simulink model "P300_directions"  (R2012b)
settings: Solver=VariableStepDiscrete  StartTime=0.0  StopTime=5000  FixedStep=1/256  RelTol=1e-3
InitFcn:
  | clear global handle
  | 
  | clear global userData
  | 
  | if exist('P300classifier') ~=1
  | global P300classifier
  | P300classifier.method = 0;
  | end
undefined symbols (not defined in the file): THblink, THfrown, THgazeL, THgazeR, THwinkL, THwinkR
libraries: dspsigops x4, dspstat3 x2, gtecHighspeedLib x2
settings Model: Creator=Markus Waldhauser  LastModifiedBy=MA
settings DataIOCC: SignalLoggingSaveFormat=ModelDataLogs
settings OptimizationCC: InitFltsAndDblsToZero=on
settings DebuggingCC: SaveWithParameterizedLinksMsg=none  SignalResolutionControl=TryResolveAllWithWarning  MultiTaskDSMMsg=warning  MultiTaskCondExecSysMsg=none  FcnCallInpInsideContextMsg=UseLocalSettings  StrictBusMsg=Warning
settings RTWCC: IncludeERTFirstTime=on
settings GRTTargetCC: TargetFcnLib=ansi_tfl_tmw.mat  CombineOutputUpdateFcns=off  GRTInterface=on

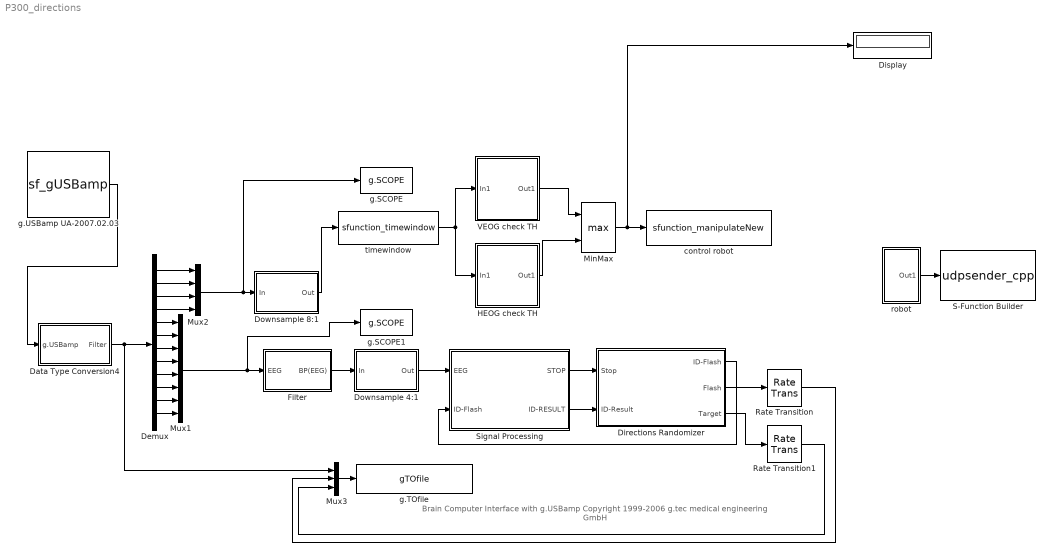
== system P300_directions ==
  note: Brain Computer Interface with g.USBamp
      | Copyright 1999-2006 g.tec medical engineering GmbH
  Data Type Conversion4 : Subsystem
  Demux : Demux  Outputs=12
  Directions Randomizer : Subsystem  mask(Single Character Flash Speller){mode=Free Ride, flashtime=100, darktime=100}
      mask prompts: flashtime "Flash time [ms]:"; darktime "Dark time [ms]:"
      mask help: Displays a 36 character matrix. Each character is flashing up for a specific time in a random and sequential order. The dark time is the time between the characters.
      mask init:
      | set_param('P300_directions/Directions Randomizer/StopSimu','Gain','0');
      | set_param('P300_directions/Directions Randomizer/Switch','Gain','0');
      mask Help:
      | Displays a 36 character matrix. Each character is flashing up for a specific time in a random and sequential order. The dark time is the time between the characters. If the character is flashing up the ID-Flash is transmitted for the Signal Processing. Flash contains the ID of every character. Target is one if a specific character for the copy spelling mode flashes up. <br><br>
      | 
      | Mode - can be Copy Spelling or Free Spelling<br><br>
      | Flash time [ms] - time that character is shown on screen <br><br>
      | Dark time [ms] - time between the characters
      mask TypeOptions mode: Copy Ride | Free Ride
      mask Display:
      | image(imread('dirs.png'))
      | port_label('output',1,'ID-Flash')
      | port_label('output',2,'Flash')
      | port_label('output',3,'Target')
      | port_label('input',1,'Stop')
      | port_label('input',2,'ID')
  Display : Display
      mask Display: disp('D blink');
  Downsample 4:1 : Subsystem
  Downsample 8:1 : Subsystem
  Filter : Subsystem  Tag=FilterWizardSubSystem
      settings: ErrorFcn=dspFilterRealizedInBasicElemsAlgLoopErrFcnCallback
  HEOG check TH : Subsystem
  MinMax : MinMax  Function=max  Inputs=2
  Mux1 : Mux  Inputs=8
  Mux2 : Mux
  Mux3 : Mux  Inputs=3
  Rate Transition : RateTransition
  Rate Transition1 : RateTransition
  S-Function Builder : S-Function  InitFcn=try, set_param(gcb,'FunctionName','udpsender_cpp'), end  FunctionName=udpsender_cpp  Parameters=int32(1)  SFunctionModules=udpsender_cpp_wrapper  EnableBusSupport=off  mask(S-Function Builder){}
      mask help: Simulink:masks:SFunctionBuilder_MD
      mask init:
      | val = [[.9  0.75 0.75 1 1 .9 .9 1]',[1 1 0.75 0.75 .9 .9 1 .9]'];try , sys = get_param(gcb,'SfunBuilderFcnName');if isempty(sys), sys = get_param(gcb,'FunctionName'); end,catch, sys = get_param(gcb,'FunctionName'); end
      settings: CopyFcn=set_param(gcbh,'LinkStatus','none')  PreSaveFcn=try, set_param(gcb,'FunctionName','udpsender_cpp'), end  OpenFcn=sfunctionwizard(gcbh)
      mask Display: plot(val(:,1),val(:,2)),disp(sys), port_label('input',1,'u0')
  Signal Processing : Subsystem  mask(P300 Signal Processing){windTime=800, runmax=2, channels=8, method=Linear Discriminant Analysis}
      mask prompts: windTime "Buffer length [ms]"; runmax "Number of flashes:"; channels "Number of channels:"; method "Classification Method:"
      mask help: The block buffers EEG data for each ID-Flash obtained. As soon as M (Number of flashes) characters of each ID are obtained a STOP command is sent and the maximum P300 is calculated and applied on output ID.
      mask Help:
      | P300 Signal Processing block. The block buffers EEG data for each ID-Flash obtained. As soon as M (Number of flashes) characters of each ID are obtained a STOP command is sent. Then the maximum P300 is calculated and the character ID is sent. <br><br>
      | 
      | Buffer length [ms] - enter the EEG data buffer size <br><br>
      | Number of flashes - enter the number each character should flash up <br><br>
      mask TypeOptions method: Linear Discriminant Analysis | Support Vector Machine
      mask Display:
      | image(imread('p3002.png'))
      | port_label('output', 1, 'STOP')
      | port_label('output', 2, 'ID')
      | port_label('input', 1, 'EEG')
      | port_label('input', 2, 'ID-Flash')
  VEOG check TH : Subsystem
  control robot : S-Function  FunctionName=sfunction_manipulateNew  EnableBusSupport=off
  g.SCOPE : gtecHighspeedLib/g.SCOPE  sdf=off
  g.SCOPE1 : gtecHighspeedLib/g.SCOPE  sdf=off
  g.TOfile : S-Function  FunctionName=gTOfile  Parameters=filename, varname, filesize, blocksize  EnableBusSupport=off  mask(g.TOfile){filename=muro_test2, varname=y, filesize=50, blocksize=1024}
      mask prompts: varname "Variable:"; filesize "File size [MB]:"; blocksize "Block size [kB]:"
      mask help:
      | The g.TOfile block saves data as a variable into a file. If you have a very large dataset, it will be splitted into more files, so it is still possible to open it in Matlab.
      |
      | Parameter:
      | Filename - name of the file, which will be extended with a four digit number
      | Variable - name of the variable, which will be extended with a four digit number
      | File size [MB] - size of the single files in megabyte
      mask Help: web(['file:///' which('gtecHS.htm')],'-helpbrowser');
      mask Callback filename:
      | set_param(gcb, 'LinkStatus', 'none');
      | maskStr = get_param(gcb, 'MaskValues');
      | tmp = sprintf('disp(''%s'')', maskStr{1});
      | set_param(gcb, 'MaskDisplay', tmp);
      | clear maskStr tmp
      mask Callback filesize:
      | maskStr = get_param(gcb, 'MaskValues');
      | mem = memory;
      | maxMem = ((mem.MaxPossibleArrayBytes*0.99)/(1024*1024));
      | if maxMem < str2num(maskStr{3})
      |     errorStr = sprintf('File size too large!\nMaximum file size: %.0f', maxMem);
      |     errordlg(errorStr);
      | end
      | clear maskStr mem maxMem errorStr
      mask Callback blocksize:
      | maskStr = get_param(gcb, 'MaskValues');
      | fileSz = str2num(maskStr{3})*1024;
      | blockSz = str2num(maskStr{4});
      | if fileSz/2 < blockSz
      |     errorStr = sprintf('Block size to large!\nMaximum half of file size');
      |     errorDlg(errorStr);
      | end
      | clear maskStr fileSz blockSz errorStr
      mask Display: disp('muro_test2')
  g.USBamp UA-2007.02.03 : S-Function  Priority=2  FunctionName=sf_gUSBamp  Parameters=cfg,snr  EnableBusSupport=off  mask{cfg=currentCFG_P300_directions_UA-2007.02.03.cfg, snr=UA-2007.02.03}
      mask prompts: cfg "Configuration"; snr "Serial"
      mask help: Enter configuration file and serial
      settings: OpenFcn=|
      | %gua_click
      | gua_block_cfg
      mask Display: image(imread('USB_symb.tif'))
  robot : Subsystem  mask{v=0.2, w=0.4, mv=stop, mw=stop, r1=off, r2=off, r3=on, r4=off, r5=off}
      mask prompts: v "linear speed"; w "angle speed"; mv "linear direction"; mw "angle  direction"; r1 "robot 1"; r2 "robot 2"; r3 "robot 3"; r4 "robot 4"; r5 "robot 5"
      mask TypeOptions mv: backward | stop | forward
      mask TypeOptions mw: right | stop | left
  timewindow : S-Function  FunctionName=sfunction_timewindow  Parameters=channel, length  EnableBusSupport=off  mask{channel=4, length=64}
      mask prompts: length "window length"
  wires:
  Data Type Conversion4/1(Filter) -> Mux3/1, Demux/1
  g.USBamp UA-2007.02.03/1 -> Data Type Conversion4/1(g.USBamp)
  Demux/1 -> Mux2/1
  Demux/2 -> Mux2/2
  Demux/3 -> Mux2/3
  Demux/4 -> Mux2/4
  Demux/5 -> Mux1/1
  Demux/6 -> Mux1/2
  Demux/7 -> Mux1/3
  Demux/8 -> Mux1/4
  Demux/9 -> Mux1/5
  Demux/10 -> Mux1/6
  Demux/11 -> Mux1/7
  Demux/12 -> Mux1/8
  Mux1/1 -> g.SCOPE1/1, Filter/1(EEG)
  Mux2/1 -> g.SCOPE/1, Downsample 8:1/1(In)
  Downsample 8:1/1(Out) -> timewindow/1
  HEOG check TH/1(Out1) -> MinMax/2
  VEOG check TH/1(Out1) -> MinMax/1
  timewindow/1 -> HEOG check TH/1(In1), VEOG check TH/1(In1)
  Filter/1(BP(EEG)) -> Downsample 4:1/1(In)
  Rate Transition/1 -> Mux3/2
  Rate Transition1/1 -> Mux3/3
  Downsample 4:1/1(Out) -> Signal Processing/1(EEG)
  Signal Processing/1(STOP) -> Directions Randomizer/1(Stop)
  Signal Processing/2(ID-RESULT) -> Directions Randomizer/2(ID-Result)
  Directions Randomizer/1(ID-Flash) -> Signal Processing/2(ID-Flash)
  Directions Randomizer/2(Flash) -> Rate Transition/1
  Directions Randomizer/3(Target) -> Rate Transition1/1
  Mux3/1 -> g.TOfile/1
  MinMax/1 -> Display/1, control robot/1
  robot/1(Out1) -> S-Function Builder/1

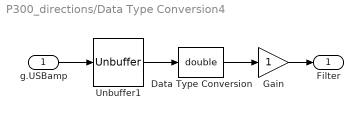
== system P300_directions/Data Type Conversion4 ==
  g.USBamp : Inport  Priority=1
  Data Type Conversion : DataTypeConversion  OutDataTypeStr=double
  Gain : Gain  SampleTime=1/256  SaturateOnIntegerOverflow=on  OutDataTypeStr=Inherit: Same as input  ParamDataTypeStr=Inherit: Same as input
  Unbuffer1 : Unbuffer
  Filter : Outport
  wires:
  Data Type Conversion/1 -> Gain/1
  Unbuffer1/1 -> Data Type Conversion/1
  Gain/1 -> Filter/1
  g.USBamp/1 -> Unbuffer1/1

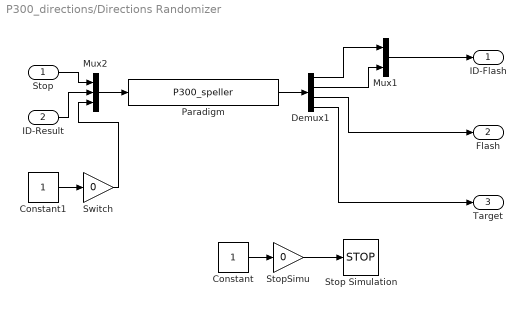
== system P300_directions/Directions Randomizer ==
  Stop : Inport
  ID-Result : Inport  Port=2
  Constant : Constant
  Constant1 : Constant
  Demux1 : Demux
  Mux1 : Mux  Inputs=2
  Mux2 : Mux  Inputs=3
  Paradigm : S-Function  FunctionName=P300_speller  Parameters=mode,flashtime,darktime  EnableBusSupport=off
  Stop Simulation : Stop
  StopSimu : Gain  Gain=0
  Switch : Gain  Gain=0  SampleTime=1/64
  ID-Flash : Outport
  Flash : Outport  Port=2
  Target : Outport  Port=3
  wires:
  Stop/1 -> Mux2/1
  ID-Result/1 -> Mux2/2
  Mux2/1 -> Paradigm/1
  Paradigm/1 -> Demux1/1
  Mux1/1 -> ID-Flash/1
  Demux1/1 -> Mux1/1
  Demux1/2 -> Mux1/2
  Demux1/3 -> Flash/1
  Demux1/4 -> Target/1
  Constant/1 -> StopSimu/1
  StopSimu/1 -> Stop Simulation/1
  Constant1/1 -> Switch/1
  Switch/1 -> Mux2/3

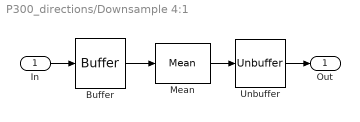
== system P300_directions/Downsample 4:1 ==
  In : Inport
  Buffer : Buffer  N=4
  Mean : dspstat3/Mean  run=off  reset_popup=None  InputProcessing=Columns as channels (frame based)  directionMode=Each column  dimension=1  treatSBRowAsCol=on  roiEnable=off  roiType=Rectangles  roiPortion=Entire ROI  roiOutput=Individual statistics for each ROI  roiFlag=off  outputDataTypeStr=Inherit: Same as accumulator  outputLastDataTypeStr=Inherit: Same as accumulator  outputMin=[]  outputMax=[]  roundingMode=Floor  overflowMode=off
  Unbuffer : Unbuffer
  Out : Outport
  wires:
  Buffer/1 -> Mean/1
  Mean/1 -> Unbuffer/1
  In/1 -> Buffer/1
  Unbuffer/1 -> Out/1

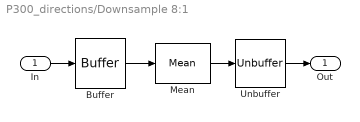
== system P300_directions/Downsample 8:1 ==
  In : Inport
  Buffer : Buffer  N=8
  Mean : dspstat3/Mean  run=off  reset_popup=None  InputProcessing=Columns as channels (frame based)  directionMode=Each column  dimension=1  treatSBRowAsCol=on  roiEnable=off  roiType=Rectangles  roiPortion=Entire ROI  roiOutput=Individual statistics for each ROI  roiFlag=off  outputDataTypeStr=Inherit: Same as accumulator  outputLastDataTypeStr=Inherit: Same as accumulator  outputMin=[]  outputMax=[]  roundingMode=Floor  overflowMode=off
  Unbuffer : Unbuffer
  Out : Outport
  wires:
  Buffer/1 -> Mean/1
  Mean/1 -> Unbuffer/1
  In/1 -> Buffer/1
  Unbuffer/1 -> Out/1

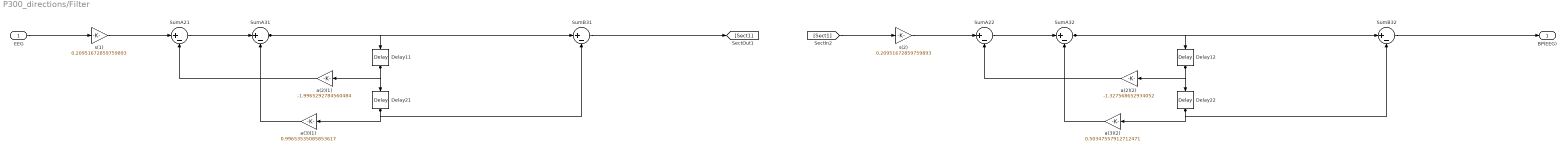
== system P300_directions/Filter ==
  EEG : Inport
  Delay{11..12,21..22} (4 alike) : dspsigops/Delay  InputProcessing=Inherited (this choice will be removed - see release notes)  dly_unit=Samples  delay=1  ic_detail=off  dif_ic_for_ch=off  dif_ic_for_dly=off  ic=0  reset_popup=None
  SumA{21..22,31..32} (4 alike) : Sum  Inputs=|+-  SaturateOnIntegerOverflow=on  InputSameDT=on  OutDataTypeStr=Inherit: Same as first input
  SumB31 : Sum  Inputs=|+-  SaturateOnIntegerOverflow=on  InputSameDT=on  OutDataTypeStr=Inherit: Same as first input
  SumB32 : Sum  Inputs=|+-  SaturateOnIntegerOverflow=on  InputSameDT=on  OutDataTypeStr=Inherit: Same as first input
  a(2)(1) : Gain  Gain=-1.9965292784560484  SaturateOnIntegerOverflow=on  OutDataTypeStr=Inherit: Same as input  ParamDataTypeStr=Inherit: Same as input
  a(2)(2) : Gain  Gain=-1.327568652934052  SaturateOnIntegerOverflow=on  OutDataTypeStr=Inherit: Same as input  ParamDataTypeStr=Inherit: Same as input
  a(3)(1) : Gain  Gain=0.99653535085853617  SaturateOnIntegerOverflow=on  OutDataTypeStr=Inherit: Same as input  ParamDataTypeStr=Inherit: Same as input
  a(3)(2) : Gain  Gain=0.50347557912712471  SaturateOnIntegerOverflow=on  OutDataTypeStr=Inherit: Same as input  ParamDataTypeStr=Inherit: Same as input
  s(1) : Gain  Gain=0.20951672859759893  SaturateOnIntegerOverflow=on  OutDataTypeStr=Inherit: Same as input  ParamDataTypeStr=Inherit: Same as input
  s(2) : Gain  Gain=0.20951672859759893  SaturateOnIntegerOverflow=on  OutDataTypeStr=Inherit: Same as input  ParamDataTypeStr=Inherit: Same as input
  BP(EEG) : Outport
  wires:
  EEG/1 -> s(1)/1
  s(1)/1 -> SumA21/1
  SumA21/1 -> SumA31/1
  SumA31/1 -> SumB31/1, Delay11/1
  SumB31/1 -> [Sect1]
  a(2)(1)/1 -> SumA21/2
  Delay11/1 -> a(2)(1)/1, Delay21/1
  a(3)(1)/1 -> SumA31/2
  Delay21/1 -> a(3)(1)/1, SumB31/2
  [Sect1] -> s(2)/1
  s(2)/1 -> SumA22/1
  SumA22/1 -> SumA32/1
  SumA32/1 -> SumB32/1, Delay12/1
  SumB32/1 -> BP(EEG)/1
  a(2)(2)/1 -> SumA22/2
  Delay12/1 -> a(2)(2)/1, Delay22/1
  a(3)(2)/1 -> SumA32/2
  Delay22/1 -> a(3)(2)/1, SumB32/2

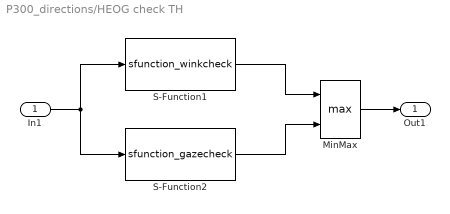
== system P300_directions/HEOG check TH ==
  In1 : Inport
  MinMax : MinMax  Function=max  Inputs=2
  S-Function1 : S-Function  FunctionName=sfunction_winkcheck  Parameters=windowlength,THL,THR  EnableBusSupport=off  mask{windowlength=24, THL=THwinkL, THR=THwinkR}
      mask prompts: windowlength "window length"; THL "threshold left"; THR "threshold right"
  S-Function2 : S-Function  FunctionName=sfunction_gazecheck  Parameters=windowlength,THL,THR  EnableBusSupport=off  mask{windowlength=16, THL=THgazeL, THR=THgazeR}
      mask prompts: windowlength "window length"; THL "threshold left"; THR "threshold right"
  Out1 : Outport
  wires:
  S-Function1/1 -> MinMax/1
  MinMax/1 -> Out1/1
  In1/1 -> S-Function2/1, S-Function1/1
  S-Function2/1 -> MinMax/2

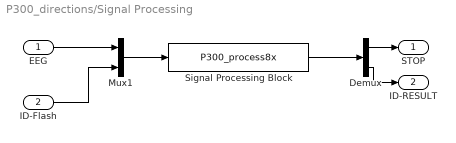
== system P300_directions/Signal Processing ==
  EEG : Inport
  ID-Flash : Inport  Port=2
  Demux : Demux  Outputs=2
  Mux1 : Mux  Inputs=2
  Signal Processing Block : S-Function  FunctionName=P300_process8x  Parameters=windTime, runmax, channels, method, P300classifier  EnableBusSupport=off
  STOP : Outport
  ID-RESULT : Outport  Port=2
  wires:
  ID-Flash/1 -> Mux1/2
  Demux/1 -> STOP/1
  Demux/2 -> ID-RESULT/1
  Mux1/1 -> Signal Processing Block/1
  Signal Processing Block/1 -> Demux/1
  EEG/1 -> Mux1/1

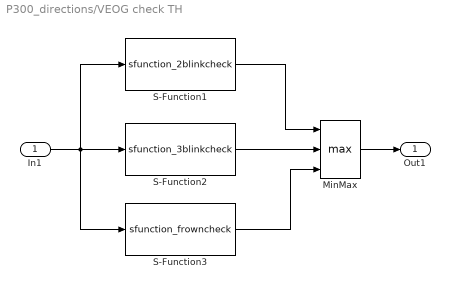
== system P300_directions/VEOG check TH ==
  In1 : Inport
  MinMax : MinMax  Function=max  Inputs=3
  S-Function1 : S-Function  FunctionName=sfunction_2blinkcheck  Parameters=windowlength,Vcl,Vop,Amin  EnableBusSupport=off  mask{windowlength=32, Vcl=THblink(1), Vop=THblink(2), Amin=THblink(3)}
      mask prompts: windowlength "window length"; Vcl "close threshold"; Vop "open threshold"; Amin "min amplitude"
  S-Function2 : S-Function  FunctionName=sfunction_3blinkcheck  Parameters=windowlength,Vcl,Vop,Amin  EnableBusSupport=off  mask{windowlength=48, Vcl=THblink(1), Vop=THblink(2), Amin=THblink(3)}
      mask prompts: windowlength "window length"; Vcl "close threshold"; Vop "open threshold"; Amin "min amplitude"
  S-Function3 : S-Function  FunctionName=sfunction_frowncheck  Parameters=windowlength,Vcl,Vop,Amin  EnableBusSupport=off  mask{windowlength=48, Vcl=THfrown(1), Vop=THfrown(2), Amin=THfrown(3)}
      mask prompts: windowlength "window length"; Vcl "close threshold"; Vop "open threshold"; Amin "min amplitude"
  Out1 : Outport
  wires:
  S-Function2/1 -> MinMax/2
  MinMax/1 -> Out1/1
  In1/1 -> S-Function3/1, S-Function2/1, S-Function1/1
  S-Function1/1 -> MinMax/1
  S-Function3/1 -> MinMax/3

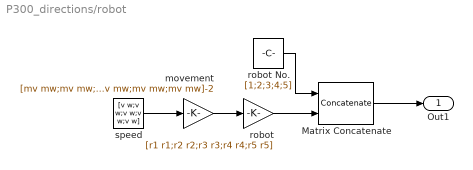
== system P300_directions/robot ==
  Matrix Concatenate : Concatenate  Mode=Multidimensional array  ConcatenateDimension=2
  movement : Gain  Gain=[mv mw;mv mw;mv mw;mv mw;mv mw]-2
  robot : Gain  Gain=[r1 r1;r2 r2;r3 r3;r4 r4;r5 r5]
  robot No. : Constant  Value=[1;2;3;4;5]  VectorParams1D=off  SampleTime=1/32
  speed : Constant  Value=[v w;v w;v w;v w;v w]  VectorParams1D=off  SampleTime=1/32
  Out1 : Outport
  wires:
  speed/1 -> movement/1
  movement/1 -> robot/1
  robot/1 -> Matrix Concatenate/2
  robot No./1 -> Matrix Concatenate/1
  Matrix Concatenate/1 -> Out1/1
